simulink model "MATE_PermanentMagnetSynchronousMachine"  (R2024b)
settings: Solver=ode5  StartTime=0.0  StopTime=1  FixedStep=Ts_sim  MaxStep=Ts_sim  MinStep=Ts_sim / 100  RelTol=1e-3
PostLoadFcn:
  | Ts_sim=1e-6; Ts=Ts_sim;T_deadtime=5e-6;
  | PMSMDrive_Param;
InitFcn:
  | Ts_sim=1e-6; Ts=Ts_sim;T_deadtime=5e-6;
  | PMSMDrive_Param;
values from neighbouring files (symbols this model uses):
  carrier = 12000    [PMSMDrive_Param.m]
  inv_id_100 = 1 / id_100    [PMSMDrive_Param.m]
  inv_iq_100 = 1 / iq_100    [PMSMDrive_Param.m]
  inv_Kt = 1 / Kt    (= 1.0729615028)    [PMSMDrive_Param.m]
  iq_100 = Irms * sqrt3    [PMSMDrive_Param.m]
  iq_max = iq_100 * Torque_Lim / 100    [PMSMDrive_Param.m]
  Jall = J1 + J2    (= 0.0167309142)    [PMSMDrive_Param.m]
  Ld_100 = Ld / 1000    (= 0.002984)    [PMSMDrive_Param.m]
  Lq_100 = Lq / 1000    (= 0.004576)    [PMSMDrive_Param.m]
  Pm = Pole / 2    (= 3)    [PMSMDrive_Param.m]
  rad_to_rpm = 60 / 2 / pi    (= 9.54929658551)    [PMSMDrive_Param.m]
  rpm_to_rad = 1 / 60 * 2 * pi    (= 0.10471975512)    [PMSMDrive_Param.m]
  tr23 = sqrt23 * [ 1 0 ; -1/2 sqrt(3)/2 ; -1/2 -sqrt(3)/2 ]    [PMSMDrive_Param.m]
  tr32 = sqrt23 * [ 1 -1/2 -1/2 ; 0 sqrt(3)/2 -sqrt(3)/2 ]    [PMSMDrive_Param.m]
  Tsc = 50e-6    (= 5e-05)    [PMSMDrive_Param.m]
  V_upper = 400    [PMSMDrive_Param.m]
  VDC = 200 * sqrt(2)    [PMSMDrive_Param.m]
  wcc = 2000    [PMSMDrive_Param.m]
  wcpi = wcc / 10    (= 200)    [PMSMDrive_Param.m]
  wsc = 200    [PMSMDrive_Param.m]
  wspi = wsc / 10    (= 20)    [PMSMDrive_Param.m]
undefined symbols (not defined in the file or in its folder): DiscIntNeverNeededParam, PMSMDrive_Param, Vf
libraries: fl_lib x15, nesl_utility x13, simetranss x8, ee_lib x6, simulink x4
settings Model: ARTEMISmethode_block_infos=$$__separator__$$  Creator=Kyle Diller  LastModifiedBy=CD8435
settings SolverCC: AlgebraicLoopSolver=TrustRegion
settings DataIOCC: LimitDataPoints=on  SaveFormat=Array  SignalLoggingSaveFormat=ModelDataLogs  ReturnWorkspaceOutputs=off
settings OptimizationCC: ExpressionDepthLimit=2147483647  InitFltsAndDblsToZero=on  LifeSpan=inf
settings DebuggingCC: AlgebraicLoopMsg=error  ArtificialAlgebraicLoopMsg=error  SaveWithParameterizedLinksMsg=none  UnderspecifiedInitializationDetection=Classic  MergeDetectMultiDrivingBlocksExec=none  SignalResolutionControl=TryResolveAllWithWarning  SolverPrmCheckMsg=warning  MultiTaskDSMMsg=warning  MultiTaskCondExecSysMsg=none  FcnCallInpInsideContextMsg=warning  UnconnectedInputMsg=warning  UnconnectedOutputMsg=warning  UnconnectedLineMsg=warning  AllowSymbolicDim=off  StateNameClashWarn=warning  SFUnexpectedBacktrackingDiag=warning  SFNoUnconditionalDefaultTransitionDiag=warning  SFExecutionAtInitializationDiag=none  ArithmeticOperatorsInVariantConditions=warning
settings HardwareCC: ProdBitPerPointer=32  ProdBitPerSizeT=32  ProdBitPerPtrDiffT=32  ProdLargestAtomicFloat=None  ProdIntDivRoundTo=Undefined  ProdEndianess=Unspecified  ProdWordSize=32  ProdHWDeviceType=32-bit Generic
settings ModelReferenceCC: EnableRefExpFcnMdlSchedulingChecks=on  PropagateSignalLabelsOutOfModel=off
settings SFSimCC: SimUseLocalCustomCode=off  CustomCodeUndefinedFunction=UseInterfaceOnly
settings RTWCC: RTWUseLocalCustomCode=off  GPUComputeCapability=3.5
settings CodeAppCC: StateflowObjectComments=on
settings GRTTargetCC: TargetFcnLib=ansi_tfl_tmw.mat  TargetLangStandard=C89/C90 (ANSI)  CombineOutputUpdateFcns=off  GRTInterface=on
settings ConfigComp: CovMetricSettings=dw  CovSaveCumulativeToWorkspaceVar=on  CovSaveSingleToWorkspaceVar=on  CovExternalEMLEnable=off
settings SimscapeCC: SimscapeNormalizeSystem=off

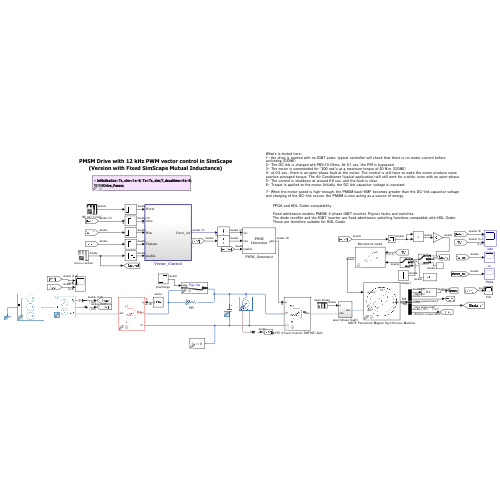
[thumbnail: Simulink's stored preview of the top-level diagram]
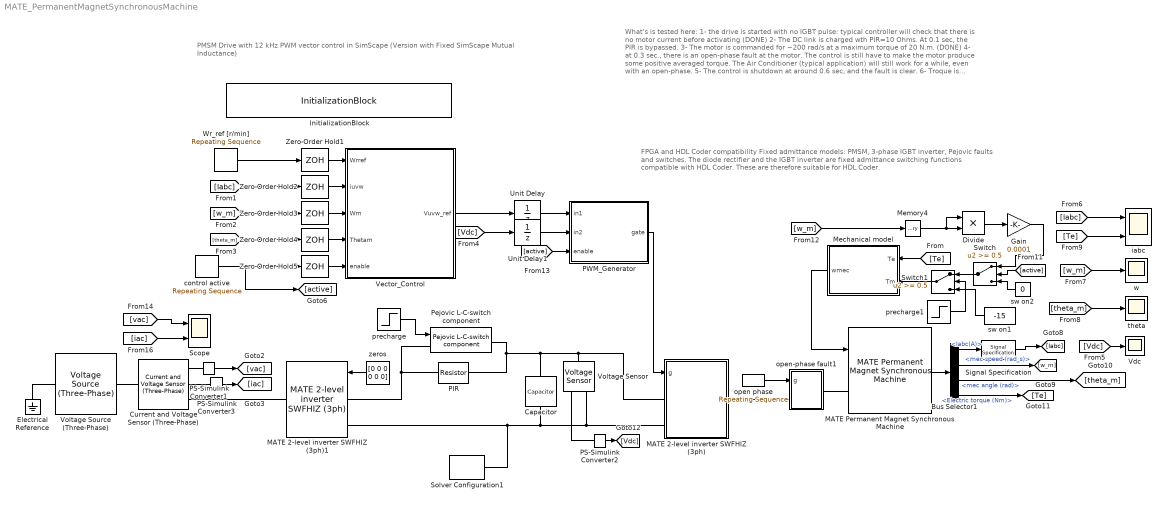
== system MATE_PermanentMagnetSynchronousMachine ==
  note: What's is tested here:
      | 1- the drive is started with no IGBT pulse: typical controller will check that there is no motor current before activating (DONE)
      | 2- The DC link is charged wth PIR=10 Ohms. At 0.1 sec, the PIR is bypassed.
      | 3- The motor is commanded for ~200 rad/s at a maximum torque of 20 N.m. (DONE)
      | 4- at 0.3 sec., there is an open-phase fault at the motor. The control is still have to make the motor produce some positive averaged torque. The Air Conditioner (typical application) will still work for a while, even with an open-phase.
      | 5- The control is shutdown at around 0.6 sec, and the fault is clear.
      | 6- Troque is applied to the motor. Initially, the DC link capacitor voltage is constant.
      |
      | 7- When the motor speed is high-enough, the PMSM back-EMF becomes greater than the DC-link capacitor voltage and charging of the DC-link occurs: the PMSM is now acting as a source of energy.
  note: PMSM Drive with 12 kHz PWM vector control in SimScape
      | (Version with Fixed SimScape Mutual Inductance)
  note: FPGA and HDL Coder compatibility
      |
      | Fixed admittance models: PMSM, 3-phase IGBT inverter, Pejovic faults and switches.
      | The diode rectifier and the IGBT inverter are fixed admittance switching functions compatible with HDL Coder.
      | These are therefore suitable for HDL Coder.
  Bus Selector1 : BusSelector  OutputSignals=Iabc(A),mec speed (rad_s),mec angle (rad),Electric torque (Nm)
  Capacitor : fl_lib/Electrical/Electrical Elements/Capacitor  c=1e-3 F  r=0 Ohm  g=0 1/Ohm  i_specify=off  i_priority=None  i=0 A  i_nominal_specify=off  i_nominal_value=1  i_nominal_unit=A  v_specify=off  v_priority=None  v=0 V  v_nominal_specify=off  v_nominal_value=1  v_nominal_unit=V  vc_specify=off  vc_priority=High  vc=0 V  vc_nominal_specify=off  vc_nominal_value=1  vc_nominal_unit=V
  Current and Voltage Sensor (Three-Phase) : ee_lib/Sensors & Transducers/Current and Voltage Sensor (Three-Phase)  vMeasurementType=ee.enum.vmeasurement.ll  outputUnit=ee.enum.unit.si  SRated=100e6 A*V  VRated=24e3 V  I_specify=off  I_priority=None  I=[0, 0, 0] A  I_nominal_specify=off  I_nominal_value=1  I_nominal_unit=A  V_specify=off  V_priority=None  V=[0, 0, 0] V  V_nominal_specify=off  V_nominal_value=1  V_nominal_unit=V
      settings: InternalSimscapePortConfiguration="{\"Bottom\":[],\"Left\":[{\"id\":\"N1\",\"label\":\"~1\",\"type\":\"foundation.electrical.three_phase\"}],\"Right\":[{\"id\":\"V_output\",\"label\":\"V\",\"type\":\"output\"},{\"id\":\"I_output\",\"label\":\"I\",\"type\":\"output\"},{\"id\":\"N2\",\"label\":\"~2\",\"type\":\"foundation.electrical.three_phase\"}],\"Top\":[]}"
  Divide : Product
  Electrical Reference : fl_lib/Electrical/Electrical Elements/Electrical Reference
  Gain : Gain  Gain=0.0001
  InitializationBlock : simetranss/Usefulls/InitializationBlock  InitVar=Ts_sim=1e-6; Ts=Ts_sim;T_deadtime=5e-6;  InitFile=PMSMDrive_Param;  prel=off  posl=on  inif=on
  MATE 2-level inverter SWFHIZ (3ph) : Subsystem  AncestorBlock=simetranss/FPGA/MATE 2-level inverter SWFHIZ (3ph)  mask(MATE Inverter Switching Function (2-level IGBT/Diode) (3-phase)){Ron=1e-3, Gpp=250, Gip=0.1e-6, Ts=Ts, min_charge=0.1}
      mask prompts: Ron "Switch Ron (Ohms)"; Gpp "Snubber resistance (Ohms)"; Gip "Snubber Capacitor (Ohms)"; Ts "Sample time (s)"; min_charge "Minimum rectifying current (A)"
      mask help:
      | This block implements a 3-phase  2-level inverter as a switching function.
      |
      | The block is Time-Step-Averaging-capable meaning that the averaging gate ON-time is averaged at each time step.
      |
      | With this approach, dead-times smaller than the sample time are accurately taken into account.
      |
      | The inverter can be in high impedance and rectifying states by selecting correctly the RC snubber.
      | Typically Rsnubber=L_load/Ts , then adjust Csnubber so Rsnubber*Csnubber=2*Ts.
      |
      | Minimum Rectifying current: In passive mode (no IGBT pulsing), this is the minimum rectifying current that is injected to the DC bus. This parameter is used to avoid unrealistic DC-bus charging when the inverter acts as a diode recfifier and do not impact in active control (gate pulsing) mode.
      |
      | The block has a constant admittance and is suitable for HDL coder.
  MATE 2-level inverter SWFHIZ (3ph)1 : simetranss/FPGA/MATE 2-level inverter SWFHIZ (3ph)  Ron=1e-3  Vf=0  Gpp=250  Gip=0.1e-6  Ts=Ts  min_charge=0.1
  MATE Permanent Magnet Synchronous Machine : simetranss/Machines/MATE Permanent Magnet Synchronous Machine  Rs=0.12  rtyp=Salient (Ld != Lq)  Ld=0.002984  Lq=0.004576  Ldd=0.003  Mf=0.25366  pp=3  AngInit=0  sal_der=0.1  Ts=Ts
  Mechanical model : Subsystem  mask(Machine rotational mechanical model){J=0.016731, F=0, fo=0, Ts=Ts}
      mask prompts: J "Inertia (kg.m^2)"; F "Friction (N.m.s)"; fo "Initial mechanical frequency (Hz)"; Ts "Sample Time (s)"
      mask help:
      | This block can implement the mechanical equation of rotating machines.
      |
      | The block working equation is:
      | wmec=1/J*INTEGRAL{( Te - Tm -F*wmec )*dt}
      |
      | All values in SI.
      |
      | Parameters:
      | Inertia J (kg.m^2)
      | Friction F (N.m.s)
      | Initial mechanical frequency (Hz)
      | Sample Time (s).
      |
      | Signals:
      | Te: electric torque input from the machine (N.m.)
      | Tm : mechanical torque applied to the shaft (N.m.)
      | wmec: mechanical speed of machine (rad/s)
      |
      | Conversion from Per-Unit values
      |
      | J=2*H*Pn/w_mec^2
      | F=D*Pn/w_mec^2
      | where:
      | J is the inertia in km.m^2
      | H is the inertia constant in seconds.
      | F is the friction factor in N.m.s
      | D in the friction factor or damping factor in pu.
      | Pn is the nominal power of the machine
      | w_mec is the nominal mechanical rotational frequency of the machine in rad/s
  Memory4 : Memory  InheritSampleTime=on
  PIR : fl_lib/Electrical/Electrical Elements/Resistor  R=10 Ohm  i_specify=off  i_priority=None  i=0 A  i_nominal_specify=off  i_nominal_value=1  i_nominal_unit=A  v_specify=off  v_priority=None  v=0 V  v_nominal_specify=off  v_nominal_value=1  v_nominal_unit=V
  PS-Simulink Converter1 : nesl_utility/PS-Simulink Converter  PhysicalDomain=network_engine_domain  SubClassName=ps_output  LeftPortType=input  RightPortType=output  PseudoPeriodic=off  Frequencies=[]  VectorFormat=inherit  Unit=inherit  AffineConversion=off
  PS-Simulink Converter2 : nesl_utility/PS-Simulink Converter  PhysicalDomain=network_engine_domain  SubClassName=ps_output  LeftPortType=input  RightPortType=output  PseudoPeriodic=off  Frequencies=[]  VectorFormat=inherit  Unit=inherit  AffineConversion=off
  PS-Simulink Converter3 : nesl_utility/PS-Simulink Converter  PhysicalDomain=network_engine_domain  SubClassName=ps_output  LeftPortType=input  RightPortType=output  PseudoPeriodic=off  Frequencies=[]  VectorFormat=inherit  Unit=inherit  AffineConversion=off
  PWM_Generator : Subsystem
      mask Display: disp(' PWM \n Generator ')
  Pejovic L-C-switch component : simetranss/FPGA/Pejovic L-C-switch component  typ=Switch  Lon=1e-7  L=100e-6  C=300e-9  traprule=off  otherSW='coming soon'  Ts=Ts  pcbp=off  showV=off  showI=off
  Scope : Scope  NumInputPorts=2
  Signal Specification : SignalSpecification  Dimensions=3
  Solver Configuration1 : nesl_utility/Solver Configuration  PhysicalDomain=network_engine_domain  SubClassName=solver  LeftPortType=input  RightPortType=generic  Tones=[]  Harmonics=[]  SimulateNoise=off  Profile=off  UseLocalSampling=off  EnableSwitchedLinearOptims=on  FrequencyDomain=off  UseCCode=off  RelTol=0.001  AbsTol=1e-06  MinStep=1e-09  ToWorkspace=off  RevertToSquareIcSolve=off  NumHomotopyIterations=100  PhasorMode=off  PhasorModeNumHarmonics=1  ConsistencySolver=NEWTON_FTOL  IndexReductionMethod=DerivativeReplacement  DoDC=off  ResidualTolerance=0.001  ConsistencyTolSource=GLOBAL  ConsistencyAbsTol=0.001  ConsistencyRelTol=0.001  ConsistencyTolFactor=0.001  UseLocalSolver=on  LocalSolverChoice=NE_BACKWARD_EULER_ADVANCER  ResolveIndetEquations=off  FunctionEvalNumThread=1  LocalSolverSampleTime=Ts  DoFixedCost=on  MaxNonlinIter=1  MaxModeIter=2  ComputeImpulses=off  ImpulseIterations=2  LinearAlgebra=Sparse  LinearAlgebraNumThread=0  EquationFormulation=NE_TIME_EF  DelaysMemoryBudget=1024  AutomaticFiltering=off  FilteringTimeConstant=0.001  PartitionStorageMethod=AS_NEEDED  PartitionMemoryBudget=1024  PartitionMethod=ROBUST  MultibodyUseLocalSolver=off  MultibodyLocalSolverChoice=ODE1  MultibodyLocalSolverSampleTime=0.001
  Switch : Switch  Threshold=0.5  SaturateOnIntegerOverflow=off  InputSameDT=off
  Switch1 : Switch  Threshold=0.5  SaturateOnIntegerOverflow=off  InputSameDT=off
  Unit Delay : UnitDelay  SampleTime=Ts  HasFrameUpgradeWarning=on
  Unit Delay1 : UnitDelay  SampleTime=Ts  HasFrameUpgradeWarning=on
  Vdc : Scope
  Vector_Control : Subsystem  TreatAsAtomicUnit=on
  Voltage Source (Three-Phase) : ee_lib/Sources/Voltage Source (Three-Phase)  vline_rms=200 V  shift=0 deg  freq=60 Hz  impedance_option=4  SShortCircuit=10000e6 A*V  XR=15  R=0.011 Ohm  L=1e-4 H  harmonic_option=0  harmonic_orders=[5, 7, 11, 13]  harmonic_ratios=[.1, .1, .1, .1]  G_parasitic=0 1/Ohm  I_specify=on  I_priority=High  I=[0, 0, 0] A  I_nominal_specify=off  I_nominal_value=1  I_nominal_unit=A
  Voltage Sensor : fl_lib/Electrical/Electrical Sensors/Voltage Sensor
  Wr_ref [r/min] : simulink/Sources/Repeating Sequence  rep_seq_t=[ 0 0.1 0.1+eps 0.15 0.15+eps 0.6]  rep_seq_y=[ 0 0 1000 1000 2000 2000] * rpm_to_rad
  Zero-Order Hold{1..5} (5 alike) : ZeroOrderHold  SampleTime=Tsc
  control active : simulink/Sources/Repeating Sequence  rep_seq_t="[ 0 0.09 0.09+Ts  0.6 0.6+Ts  2]"  rep_seq_y=[ 0 0 1 1 0 0]
  iabc : Scope  NumInputPorts=2
  open phase : simulink/Sources/Repeating Sequence  rep_seq_t="[ 0 0.4 0.4+Ts  0.6 0.6+Ts  2]"  rep_seq_y=[ 1 1 0 0 1 1]
  open-phase fault1 : Subsystem
  precharge : Step  Time=0.1  SampleTime=0
  precharge1 : Step  Time=0.7  Before=1  After=0  SampleTime=0
  sw on1 : Constant  Value=-15
  sw on2 : Constant  Value=0
  theta : Scope
  w : Scope
  zeros : Constant  Value=[0 0 0 0 0 0]
  wires:
  [theta_m] -> Zero-Order Hold4/1
  [w_m] -> Zero-Order Hold3/1
  [Iabc] -> Zero-Order Hold2/1
  [w_m] -> Memory4/1
  Wr_ref [r/min]/1 -> Zero-Order Hold1/1
  Vector_Control/1(Vuvw_ref) -> Unit Delay/1
  [Vdc] -> Unit Delay1/1
  [Vdc] -> Vdc/1
  [Iabc] -> iabc/1
  [w_m] -> w/1
  [theta_m] -> theta/1
  [Te] -> iabc/2
  control active/1 -> [active], Zero-Order Hold5/1
  [active] -> Switch/2
  [active] -> PWM_Generator/3(enable)
  [Te] -> Mechanical model/1(Te)
  PWM_Generator/1(gate) -> MATE 2-level inverter SWFHIZ (3ph)/1(g)
  Bus Selector1/3 -> [theta_m]  "<mec angle (rad)>"
  Bus Selector1/2 -> [w_m]  "<mec speed (rad_s)>"
  Bus Selector1/4 -> [Te]  "<Electric torque (Nm)>"
  Bus Selector1/1 -> Signal Specification/1  "<Iabc(A)>"
  PS-Simulink Converter2/1 -> [Vdc]
  Zero-Order Hold1/1 -> Vector_Control/1(Wrref)
  Zero-Order Hold2/1 -> Vector_Control/2(iuvw)
  Zero-Order Hold3/1 -> Vector_Control/3(Wm)
  Zero-Order Hold4/1 -> Vector_Control/4(Thetam)
  Zero-Order Hold5/1 -> Vector_Control/5(enable)
  Unit Delay/1 -> PWM_Generator/1(in1)
  open phase/1 -> open-phase fault1/1(g)
  precharge/1 -> Pejovic L-C-switch component/1
  Mechanical model/1(wmec) -> MATE Permanent Magnet Synchronous Machine/1
  sw on1/1 -> Switch1/3
  precharge1/1 -> Switch1/2
  Unit Delay1/1 -> PWM_Generator/2(in2)
  PS-Simulink Converter1/1 -> [vac]
  PS-Simulink Converter3/1 -> [iac]
  [vac] -> Scope/1
  [iac] -> Scope/2
  sw on2/1 -> Switch/3
  Memory4/1 -> Divide/1, Divide/2
  Divide/1 -> Gain/1
  Gain/1 -> Switch/1
  zeros/1 -> MATE 2-level inverter SWFHIZ (3ph)1/1
  Switch1/1 -> Mechanical model/2(Tm)
  Switch/1 -> Switch1/1
  Signal Specification/1 -> [Iabc]
  MATE Permanent Magnet Synchronous Machine/1 -> Bus Selector1/1
  connections:
  Electrical Reference/LConn1 -- Voltage Source (Three-Phase)/LConn1
  Pejovic L-C-switch component/RConn1 -- PIR/RConn1 -- Capacitor/LConn1 -- Voltage Sensor/LConn1 -- MATE 2-level inverter SWFHIZ (3ph)/LConn1
  Capacitor/RConn1 -- Voltage Sensor/RConn2 -- MATE 2-level inverter SWFHIZ (3ph)/LConn2 -- Solver Configuration1/RConn1 -- MATE 2-level inverter SWFHIZ (3ph)1/LConn2
  Voltage Sensor/RConn1 -- PS-Simulink Converter2/LConn1
  Voltage Source (Three-Phase)/RConn1 -- Current and Voltage Sensor (Three-Phase)/LConn1
  MATE 2-level inverter SWFHIZ (3ph)1/RConn1 -- Current and Voltage Sensor (Three-Phase)/RConn3
  PS-Simulink Converter1/LConn1 -- Current and Voltage Sensor (Three-Phase)/RConn1
  Current and Voltage Sensor (Three-Phase)/RConn2 -- PS-Simulink Converter3/LConn1
  MATE 2-level inverter SWFHIZ (3ph)1/LConn1 -- PIR/LConn1 -- Pejovic L-C-switch component/LConn1
  MATE Permanent Magnet Synchronous Machine/LConn1 -- open-phase fault1/RConn1
  MATE 2-level inverter SWFHIZ (3ph)/RConn1 -- open-phase fault1/LConn1

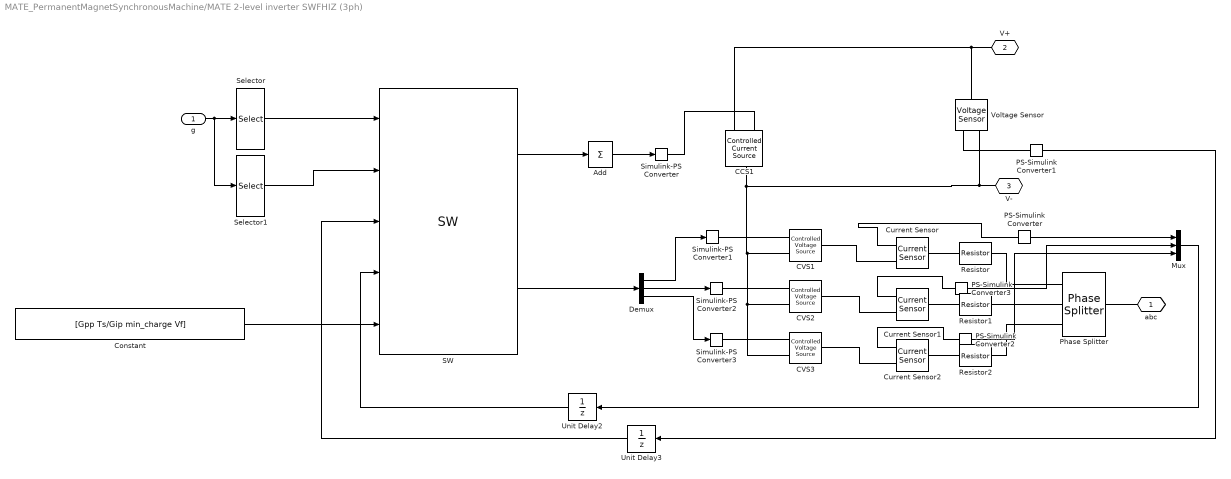
== system MATE_PermanentMagnetSynchronousMachine/MATE 2-level inverter SWFHIZ (3ph) ==
  g : Inport
  Add : Sum  Inputs=+
  CCS1 : fl_lib/Electrical/Electrical Sources/Controlled Current Source
  CVS1 : fl_lib/Electrical/Electrical Sources/Controlled Voltage Source
  CVS2 : fl_lib/Electrical/Electrical Sources/Controlled Voltage Source
  CVS3 : fl_lib/Electrical/Electrical Sources/Controlled Voltage Source
  Constant : Constant  Value=[Gpp Ts/Gip min_charge Vf]
  Current Sensor : fl_lib/Electrical/Electrical Sensors/Current Sensor
  Current Sensor1 : fl_lib/Electrical/Electrical Sensors/Current Sensor
  Current Sensor2 : fl_lib/Electrical/Electrical Sensors/Current Sensor
  Demux : Demux  Outputs=3
  Mux : Mux  Inputs=3
  PS-Simulink Converter{,1..3} (4 alike) : nesl_utility/PS-Simulink Converter  PhysicalDomain=network_engine_domain  SubClassName=ps_output  LeftPortType=input  RightPortType=output  PseudoPeriodic=off  Frequencies=[]  VectorFormat=inherit  Unit=inherit  AffineConversion=off
  Phase Splitter : ee_lib/Connectors & References/Phase Splitter
  Resistor : fl_lib/Electrical/Electrical Elements/Resistor  R=Ron Ohm  i_specify=off  i_priority=None  i=0 A  i_nominal_specify=off  i_nominal_value=1  i_nominal_unit=A  v_specify=off  v_priority=None  v=0 V  v_nominal_specify=off  v_nominal_value=1  v_nominal_unit=V
  Resistor1 : fl_lib/Electrical/Electrical Elements/Resistor  R=Ron Ohm  i_specify=off  i_priority=None  i=0 A  i_nominal_specify=off  i_nominal_value=1  i_nominal_unit=A  v_specify=off  v_priority=None  v=0 V  v_nominal_specify=off  v_nominal_value=1  v_nominal_unit=V
  Resistor2 : fl_lib/Electrical/Electrical Elements/Resistor  R=Ron Ohm  i_specify=off  i_priority=None  i=0 A  i_nominal_specify=off  i_nominal_value=1  i_nominal_unit=A  v_specify=off  v_priority=None  v=0 V  v_nominal_specify=off  v_nominal_value=1  v_nominal_unit=V
  SW : simetranss/FPGA/MATE 2-level inverter SWFHIZ/SW  SystemSampleTime=-1  VariantActivationTime=update diagram  AllowFlexibleInterface=on  Latency=0  AutoFrameSizeCalculation=off
  Selector : Selector  InputPortWidth=6  IndexOptions=Index vector (dialog)  Indices=[1 3 5]  OutputSizes=1
  Selector1 : Selector  InputPortWidth=6  IndexOptions=Index vector (dialog)  Indices=[1 3 5]+1  OutputSizes=1
  Simulink-PS Converter{,1..3} (4 alike) : nesl_utility/Simulink-PS Converter  PhysicalDomain=network_engine_domain  SubClassName=ps_input  LeftPortType=input  RightPortType=output  PseudoPeriodic=off  Frequencies=[]  NoiseDistribution=none  NoiseParameters=[]  Unit=1  AffineConversion=off  FilteringAndDerivatives=provide  SimscapeFilterOrder=1  InputFilterTimeConstant=0.001  UdotUserProvided=0
  Unit Delay2 : UnitDelay  SampleTime=Ts  HasFrameUpgradeWarning=on
  Unit Delay3 : UnitDelay  SampleTime=Ts  HasFrameUpgradeWarning=on
  Voltage Sensor : fl_lib/Electrical/Electrical Sensors/Voltage Sensor
  abc : PMIOPort  Side=Right
  V+ : PMIOPort  Port=2  Side=Left
  V- : PMIOPort  Port=3  Side=Left
  wires:
  Add/1 -> Simulink-PS Converter/1
  g/1 -> Selector1/1, Selector/1
  SW/1 -> Add/1
  PS-Simulink Converter/1 -> Mux/1
  PS-Simulink Converter3/1 -> Mux/2
  PS-Simulink Converter2/1 -> Mux/3
  Demux/3 -> Simulink-PS Converter3/1
  Demux/2 -> Simulink-PS Converter2/1
  Demux/1 -> Simulink-PS Converter1/1
  SW/2 -> Demux/1
  Selector/1 -> SW/1
  Selector1/1 -> SW/2
  Constant/1 -> SW/5
  PS-Simulink Converter1/1 -> Unit Delay3/1
  Mux/1 -> Unit Delay2/1
  Unit Delay2/1 -> SW/4
  Unit Delay3/1 -> SW/3
  connections:
  Simulink-PS Converter/RConn1 -- CCS1/RConn1
  PS-Simulink Converter/LConn1 -- Current Sensor/RConn1
  Simulink-PS Converter1/RConn1 -- CVS1/RConn1
  CVS1/RConn2 -- V-/RConn1 -- Voltage Sensor/RConn2 -- CCS1/LConn1 -- CVS2/RConn2 -- CVS3/RConn2
  CCS1/RConn2 -- V+/RConn1 -- Voltage Sensor/LConn1
  PS-Simulink Converter1/LConn1 -- Voltage Sensor/RConn1
  Phase Splitter/LConn1 -- abc/RConn1
  Resistor/RConn1 -- Phase Splitter/RConn1
  Resistor1/RConn1 -- Phase Splitter/RConn2
  Resistor2/RConn1 -- Phase Splitter/RConn3
  PS-Simulink Converter3/LConn1 -- Current Sensor1/RConn1
  PS-Simulink Converter2/LConn1 -- Current Sensor2/RConn1
  Simulink-PS Converter2/RConn1 -- CVS2/RConn1
  Simulink-PS Converter3/RConn1 -- CVS3/RConn1
  CVS1/LConn1 -- Current Sensor/RConn2
  CVS2/LConn1 -- Current Sensor1/RConn2
  CVS3/LConn1 -- Current Sensor2/RConn2
  Current Sensor2/LConn1 -- Resistor2/LConn1
  Current Sensor1/LConn1 -- Resistor1/LConn1
  Current Sensor/LConn1 -- Resistor/LConn1

== system MATE_PermanentMagnetSynchronousMachine/Mechanical model ==
  note: Pm=Tm*w so a divider by w can be added if Pm is provided instead of Tm
  Te : Inport  PortDimensions=1
  Tm : Inport  Port=2
  1 ----- J : Gain  Gain=1/J  SaturateOnIntegerOverflow=on  OutDataTypeStr=Inherit: Same as input  ParamDataTypeStr=Inherit: Same as input
  F : Gain  Gain=F  SaturateOnIntegerOverflow=on  OutDataTypeStr=Inherit: Same as input  ParamDataTypeStr=Inherit: Same as input
  Rotor speed interator : DiscreteIntegrator  InitialCondition=fo*2*pi  SampleTime=Ts  ICPrevOutput=DiscIntNeverNeededParam  ICPrevScaledInput=DiscIntNeverNeededParam
  Sum2 : Sum  Inputs=-+-  InputSameDT=on  SaturateOnIntegerOverflow=on  OutDataTypeStr=Inherit: Same as first input
  wmec : Outport  InitialOutput=0  VectorParamsAs1DForOutWhenUnconnected=off
  wires:
  Tm/1 -> Sum2/1  "Tm"
  Sum2/1 -> 1 ----- J/1
  F/1 -> Sum2/3
  Te/1 -> Sum2/2  "Te"
  1 ----- J/1 -> Rotor speed interator/1
  Rotor speed interator/1 -> wmec/1, F/1  "w"

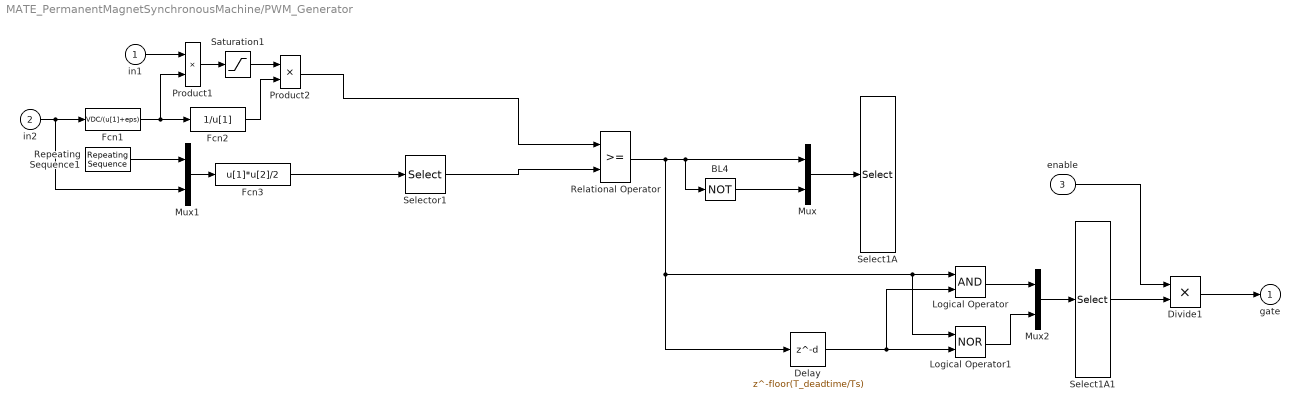
== system MATE_PermanentMagnetSynchronousMachine/PWM_Generator ==
  in1 : Inport
  in2 : Inport  Port=2
  enable : Inport  Port=3
  BL4 : Logic  Operator=NOT  Inputs=1
  Delay : Delay  DelayLength=floor(T_deadtime/Ts)
  Divide1 : Product
  Fcn1 : Fcn  Expr=VDC/(u[1]+eps)
  Fcn2 : Fcn  Expr=1/u[1]
  Fcn3 : Fcn  Expr=u[1]*u[2]/2
  Logical Operator : Logic  AllPortsSameDT=off  OutDataTypeStr=boolean
  Logical Operator1 : Logic  Operator=NOR  AllPortsSameDT=off  OutDataTypeStr=boolean
  Mux : Mux  Inputs=2
  Mux1 : Mux  Inputs=2
  Mux2 : Mux  Inputs=2
  Product1 : Product  InputSameDT=on  SaturateOnIntegerOverflow=on  OutDataTypeStr=Inherit: Same as first input
  Product2 : Product  InputSameDT=on  SaturateOnIntegerOverflow=on  OutDataTypeStr=Inherit: Same as first input
  Relational Operator : RelationalOperator
  Repeating Sequence1 : simulink/Sources/Repeating Sequence  rep_seq_t=[ 0 1/carrier/2 1/carrier ]  rep_seq_y=[ -1 1 -1 ]
  Saturation1 : Saturate  UpperLimit=VDC/2  LowerLimit=-VDC/2
  Select1A : Selector  InputPortWidth=6  IndexOptions=Index vector (dialog)  Indices=[1 4 2 5 3 6]  OutputSizes=1
  Select1A1 : Selector  InputPortWidth=6  IndexOptions=Index vector (dialog)  Indices=[1 4 2 5 3 6]  OutputSizes=1
  Selector1 : Selector  InputPortWidth=1  IndexOptions=Index vector (dialog)  Indices=[1 1 1]  OutputSizes=1
  gate : Outport  VectorParamsAs1DForOutWhenUnconnected=off
  wires:
  Selector1/1 -> Relational Operator/2
  Repeating Sequence1/1 -> Mux1/1
  Mux1/1 -> Fcn3/1
  Fcn2/1 -> Product2/2
  Saturation1/1 -> Product2/1
  Product1/1 -> Saturation1/1
  Fcn1/1 -> Fcn2/1, Product1/2
  in1/1 -> Product1/1
  Product2/1 -> Relational Operator/1
  in2/1 -> Fcn1/1, Mux1/2
  Fcn3/1 -> Selector1/1
  Relational Operator/1 -> Delay/1, Logical Operator1/1, Logical Operator/1, BL4/1, Mux/1
  BL4/1 -> Mux/2
  Mux/1 -> Select1A/1
  enable/1 -> Divide1/1
  Delay/1 -> Logical Operator/2, Logical Operator1/2
  Logical Operator/1 -> Mux2/1
  Logical Operator1/1 -> Mux2/2
  Mux2/1 -> Select1A1/1
  Select1A1/1 -> Divide1/2
  Divide1/1 -> gate/1

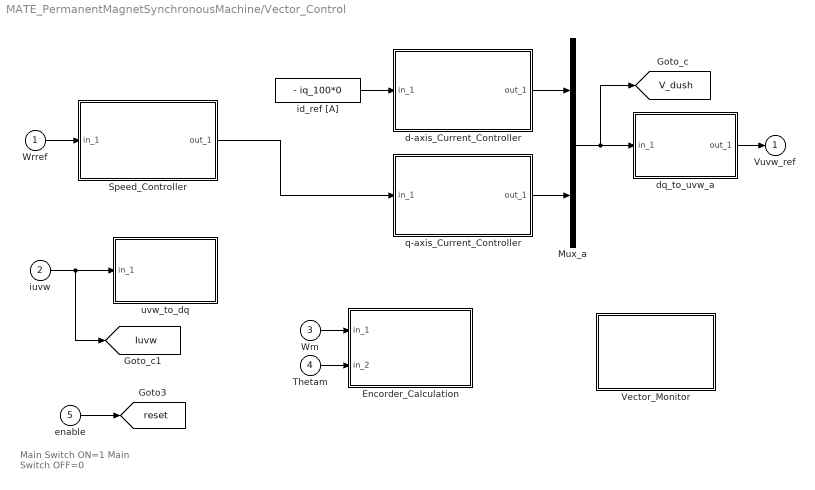
== system MATE_PermanentMagnetSynchronousMachine/Vector_Control ==
  note: Main Switch ON=1
      | Main Switch OFF=0
  Wrref : Inport
  iuvw : Inport  Port=2
  Wm : Inport  Port=3
  Thetam : Inport  Port=4
  enable : Inport  Port=5
  Encorder_Calculation : Subsystem
      mask Display: disp(' Encorder \n Calculation ')
  Mux_a : Mux  Inputs=2
  Speed_Controller : Subsystem
      mask Display: disp(' Speed \n Controller ')
  Vector_Monitor : Subsystem
      mask Display:
      | plot([0,1],[0,0])
      | plot([0,1],[1,1])
      | disp(' Vector \n Monitor ')
  d-axis_Current_Controller : Subsystem
      mask Display: disp(' Current \n Controller ')
  dq_to_uvw_a : Subsystem
      mask Display: disp(' Coordinate \n Transform')
  id_ref [A] : Constant  Value=- iq_100*0
  q-axis_Current_Controller : Subsystem
      mask Display: disp(' Current \n Controller ')
  uvw_to_dq : Subsystem
      mask Display: disp(' Coordinate \n Transform ')
  Vuvw_ref : Outport  InitialOutput=0
  tag scope: Iuvw=global, V_dush=global, reset=global
  wires:
  Wrref/1 -> Speed_Controller/1(in_1)
  Wm/1 -> Encorder_Calculation/1(in_1)
  iuvw/1 -> uvw_to_dq/1(in_1), [Iuvw]
  q-axis_Current_Controller/1(out_1) -> Mux_a/2
  d-axis_Current_Controller/1(out_1) -> Mux_a/1
  Mux_a/1 -> dq_to_uvw_a/1(in_1), [V_dush]
  dq_to_uvw_a/1(out_1) -> Vuvw_ref/1
  Thetam/1 -> Encorder_Calculation/2(in_2)
  enable/1 -> [reset]
  Speed_Controller/1(out_1) -> q-axis_Current_Controller/1(in_1)
  id_ref [A]/1 -> d-axis_Current_Controller/1(in_1)

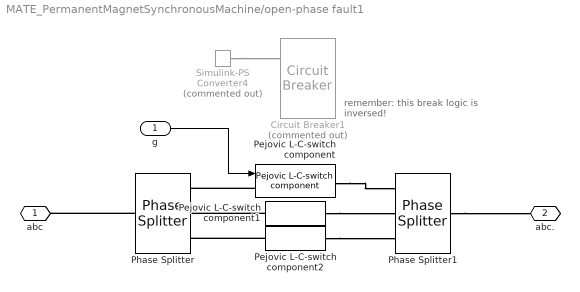
== system MATE_PermanentMagnetSynchronousMachine/open-phase fault1 ==
  note: remember: this break logic is inversed!
  g : Inport
  Circuit Breaker1 : ee_lib/Switches & Breakers/Circuit Breaker  Commented=on  R_closed=0.01 Ohm  G_open=1e-6 1/Ohm  threshold=0.5 V  breaker_behavior=ee.enum.switches.breakerBehavior.zeroCrossingDisable
      settings: InternalSimscapePortConfiguration="{\"Bottom\":[],\"Left\":[{\"id\":\"vT\",\"label\":\"vT\",\"type\":\"input\"},{\"id\":\"p1\",\"label\":\"\",\"type\":\"foundation.electrical.electrical\"}],\"Right\":[{\"id\":\"p2\",\"label\":\"\",\"type\":\"foundation.electrical.electrical\"}],\"Top\":[]}"
  Pejovic L-C-switch component : simetranss/FPGA/Pejovic L-C-switch component  typ=Switch  Lon=1e-7  L=100e-6  C=300e-9  traprule=off  otherSW='coming soon'  Ts=Ts  pcbp=off  showV=off  showI=off
  Pejovic L-C-switch component1 : simetranss/FPGA/Pejovic L-C-switch component  typ=Inductor  Lon=1e-7  L=1e-7  C=300e-9  traprule=off  otherSW='coming soon'  Ts=Ts  pcbp=off  showV=off  showI=off
  Pejovic L-C-switch component2 : simetranss/FPGA/Pejovic L-C-switch component  typ=Inductor  Lon=1e-7  L=1e-7  C=300e-9  traprule=off  otherSW='coming soon'  Ts=Ts  pcbp=off  showV=off  showI=off
  Phase Splitter : ee_lib/Connectors & References/Phase Splitter
  Phase Splitter1 : ee_lib/Connectors & References/Phase Splitter
  Simulink-PS Converter4 : nesl_utility/Simulink-PS Converter  Commented=on  PhysicalDomain=network_engine_domain  SubClassName=ps_input  LeftPortType=input  RightPortType=output  PseudoPeriodic=off  Frequencies=[]  NoiseDistribution=none  NoiseParameters=[]  Unit=1  AffineConversion=off  FilteringAndDerivatives=provide  SimscapeFilterOrder=1  InputFilterTimeConstant=0.001  UdotUserProvided=0
  abc : PMIOPort  Side=Left
  abc. : PMIOPort  Port=2  Side=Right
  wires:
  g/1 -> Pejovic L-C-switch component/1
  connections:
  Pejovic L-C-switch component2/RConn1 -- Phase Splitter1/RConn3
  Pejovic L-C-switch component1/RConn1 -- Phase Splitter1/RConn2
  Simulink-PS Converter4/RConn1 -- Circuit Breaker1/LConn1
  Phase Splitter1/LConn1 -- abc./RConn1
  Pejovic L-C-switch component1/LConn1 -- Phase Splitter/RConn2
  Phase Splitter/LConn1 -- abc/RConn1
  Pejovic L-C-switch component/RConn1 -- Phase Splitter1/RConn1
  Pejovic L-C-switch component2/LConn1 -- Phase Splitter/RConn3
  Pejovic L-C-switch component/LConn1 -- Phase Splitter/RConn1

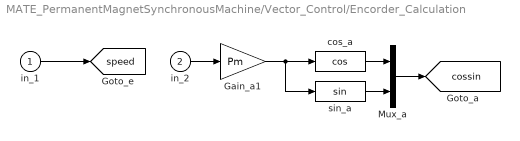
== system MATE_PermanentMagnetSynchronousMachine/Vector_Control/Encorder_Calculation ==
  in_1 : Inport
  in_2 : Inport  Port=2
  Gain_a1 : Gain  Gain=Pm  SaturateOnIntegerOverflow=on  OutDataTypeStr=Inherit: Same as input  ParamDataTypeStr=Inherit: Same as input
  Mux_a : Mux  Inputs=2
  cos_a : Trigonometry  Operator=cos
  sin_a : Trigonometry
  tag scope: cossin=global, speed=global
  wires:
  Mux_a/1 -> [cossin]
  sin_a/1 -> Mux_a/2
  cos_a/1 -> Mux_a/1
  in_2/1 -> Gain_a1/1
  in_1/1 -> [speed]
  Gain_a1/1 -> cos_a/1, sin_a/1

== system MATE_PermanentMagnetSynchronousMachine/Vector_Control/Speed_Controller ==
  in_1 : Inport
  PI_Controller : Subsystem
      mask Display: disp(' PI \n Controller ')
  error : Subsystem
      mask Display: disp('err')
  out_1 : Outport
  wires:
  error/1(out_1) -> PI_Controller/1(in_1)
  PI_Controller/1(out_1) -> out_1/1
  in_1/1 -> error/1(in_1)
  [speed] -> error/2(in_2)

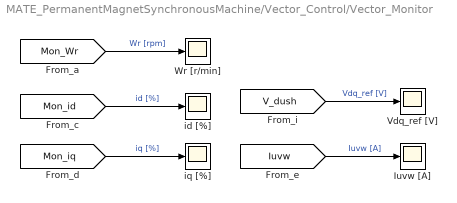
== system MATE_PermanentMagnetSynchronousMachine/Vector_Control/Vector_Monitor ==
  Iuvw [A] : Scope
  Vdq_ref [V] : Scope
  Wr [r/min] : Scope
  id [%] : Scope
  iq [%] : Scope
  wires:
  [Mon_iq] -> iq [%]/1  "iq [%]"
  [Mon_id] -> id [%]/1  "id [%]"
  [Mon_Wr] -> Wr [r/min]/1  "Wr [rpm]"
  [Iuvw] -> Iuvw [A]/1  "Iuvw [A]"
  [V_dush] -> Vdq_ref [V]/1  "Vdq_ref [V]"

== system MATE_PermanentMagnetSynchronousMachine/Vector_Control/d-axis_Current_Controller ==
  in_1 : Inport
  PI_Controller : Subsystem
      mask Display: disp(' PI \n Controller ')
  error : Subsystem
      mask Display: disp('err')
  out_1 : Outport
  wires:
  error/1(out_1) -> PI_Controller/1(in_1)
  PI_Controller/1(out_1) -> out_1/1
  in_1/1 -> error/1(in_1)
  [id_FB] -> error/2(in_2)

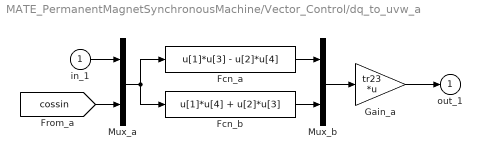
== system MATE_PermanentMagnetSynchronousMachine/Vector_Control/dq_to_uvw_a ==
  in_1 : Inport
  Fcn_a : Fcn  Expr=u[1]*u[3] - u[2]*u[4]
  Fcn_b : Fcn  Expr=u[1]*u[4] + u[2]*u[3]
  Gain_a : Gain  Gain=tr23  Multiplication=Matrix(K*u)  SaturateOnIntegerOverflow=on  OutDataTypeStr=Inherit: Same as input  ParamDataTypeStr=Inherit: Same as input
  Mux_a : Mux  Inputs=2
  Mux_b : Mux  Inputs=2
  out_1 : Outport
  wires:
  Mux_b/1 -> Gain_a/1
  Fcn_b/1 -> Mux_b/2
  Fcn_a/1 -> Mux_b/1
  Gain_a/1 -> out_1/1
  in_1/1 -> Mux_a/1
  [cossin] -> Mux_a/2
  Mux_a/1 -> Fcn_a/1, Fcn_b/1

== system MATE_PermanentMagnetSynchronousMachine/Vector_Control/q-axis_Current_Controller ==
  in_1 : Inport
  PI_Controller : Subsystem
      mask Display: disp(' PI \n Controller ')
  error : Subsystem
      mask Display: disp('err')
  out_1 : Outport
  wires:
  [iq_FB] -> error/2(in_2)
  in_1/1 -> error/1(in_1)
  PI_Controller/1(out_1) -> out_1/1
  error/1(out_1) -> PI_Controller/1(in_1)

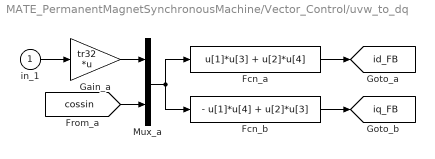
== system MATE_PermanentMagnetSynchronousMachine/Vector_Control/uvw_to_dq ==
  in_1 : Inport
  Fcn_a : Fcn  Expr=u[1]*u[3] + u[2]*u[4]
  Fcn_b : Fcn  Expr=- u[1]*u[4] + u[2]*u[3]
  Gain_a : Gain  Gain=tr32  Multiplication=Matrix(K*u)  SaturateOnIntegerOverflow=on  OutDataTypeStr=Inherit: Same as input  ParamDataTypeStr=Inherit: Same as input
  Mux_a : Mux  Inputs=2
  tag scope: id_FB=global, iq_FB=global
  wires:
  Gain_a/1 -> Mux_a/1
  in_1/1 -> Gain_a/1
  [cossin] -> Mux_a/2
  Mux_a/1 -> Fcn_a/1, Fcn_b/1
  Fcn_b/1 -> [iq_FB]
  Fcn_a/1 -> [id_FB]

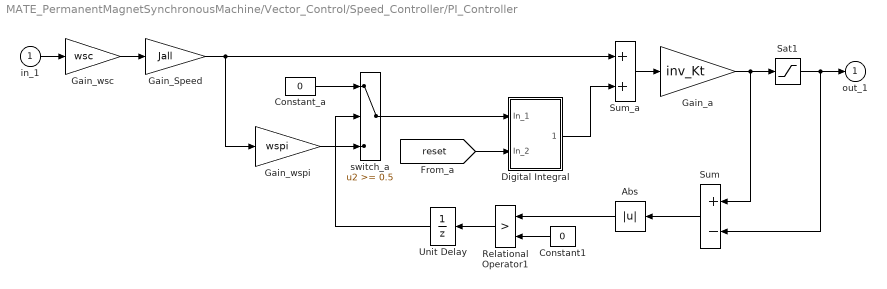
== system MATE_PermanentMagnetSynchronousMachine/Vector_Control/Speed_Controller/PI_Controller ==
  in_1 : Inport
  Abs : Abs  SaturateOnIntegerOverflow=off
  Constant1 : Constant  Value=0
  Constant_a : Constant  Value=0
  Digital Integral : Subsystem
      mask Display: disp(' 1 \n -- \n s ')
  Gain_Speed : Gain  Gain=Jall  SaturateOnIntegerOverflow=on  OutDataTypeStr=Inherit: Same as input  ParamDataTypeStr=Inherit: Same as input
  Gain_a : Gain  Gain=inv_Kt  SaturateOnIntegerOverflow=on  OutDataTypeStr=Inherit: Same as input  ParamDataTypeStr=Inherit: Same as input
  Gain_wsc : Gain  Gain=wsc  SaturateOnIntegerOverflow=on  OutDataTypeStr=Inherit: Same as input  ParamDataTypeStr=Inherit: Same as input
  Gain_wspi : Gain  Gain=wspi  SaturateOnIntegerOverflow=on  OutDataTypeStr=Inherit: Same as input  ParamDataTypeStr=Inherit: Same as input
  Relational Operator1 : RelationalOperator  Operator=>  InputSameDT=off
  Sat1 : Saturate  UpperLimit=iq_max  LowerLimit=-iq_max
  Sum : Sum  Inputs=+-  InputSameDT=on  SaturateOnIntegerOverflow=on  OutDataTypeStr=Inherit: Same as first input
  Sum_a : Sum  InputSameDT=on  SaturateOnIntegerOverflow=on  OutDataTypeStr=Inherit: Same as first input
  Unit Delay : UnitDelay  SampleTime=-1  HasFrameUpgradeWarning=on
  switch_a : Switch  Threshold=0.5
  out_1 : Outport
  wires:
  Gain_wspi/1 -> switch_a/3
  Gain_wsc/1 -> Gain_Speed/1
  in_1/1 -> Gain_wsc/1
  Constant_a/1 -> switch_a/1
  Gain_Speed/1 -> Gain_wspi/1, Sum_a/1
  switch_a/1 -> Digital Integral/1(In_1)
  [reset] -> Digital Integral/2(In_2)
  Digital Integral/1(Out_1) -> Sum_a/2
  Sum_a/1 -> Gain_a/1
  Gain_a/1 -> Sat1/1, Sum/1
  Constant1/1 -> Relational Operator1/2
  Sum/1 -> Abs/1
  Relational Operator1/1 -> Unit Delay/1
  Sat1/1 -> out_1/1, Sum/2
  Unit Delay/1 -> switch_a/2
  Abs/1 -> Relational Operator1/1

== system MATE_PermanentMagnetSynchronousMachine/Vector_Control/Speed_Controller/error ==
  in_1 : Inport
  in_2 : Inport  Port=2
  Mux_a : Mux  Inputs=2
  Sum_a : Sum  Inputs=+-  InputSameDT=on  SaturateOnIntegerOverflow=on  OutDataTypeStr=Inherit: Same as first input
  gain_a : Gain  Gain=rad_to_rpm  SaturateOnIntegerOverflow=on  OutDataTypeStr=Inherit: Same as input  ParamDataTypeStr=Inherit: Same as input
  out_1 : Outport
  tag scope: Mon_Wr=global
  wires:
  Sum_a/1 -> out_1/1
  in_2/1 -> Mux_a/2, Sum_a/2
  in_1/1 -> Sum_a/1, Mux_a/1
  Mux_a/1 -> gain_a/1
  gain_a/1 -> [Mon_Wr]

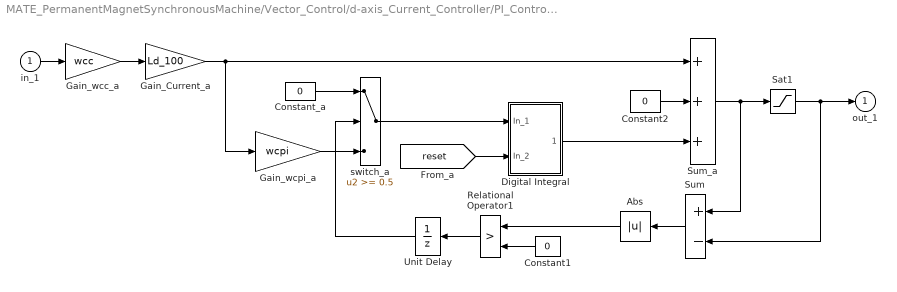
== system MATE_PermanentMagnetSynchronousMachine/Vector_Control/d-axis_Current_Controller/PI_Controller ==
  in_1 : Inport
  Abs : Abs  SaturateOnIntegerOverflow=off
  Constant1 : Constant  Value=0
  Constant2 : Constant  Value=0
  Constant_a : Constant  Value=0
  Digital Integral : Subsystem
      mask Display: disp(' 1 \n -- \n s ')
  Gain_Current_a : Gain  Gain=Ld_100  SaturateOnIntegerOverflow=on  OutDataTypeStr=Inherit: Same as input  ParamDataTypeStr=Inherit: Same as input
  Gain_wcc_a : Gain  Gain=wcc  SaturateOnIntegerOverflow=on  OutDataTypeStr=Inherit: Same as input  ParamDataTypeStr=Inherit: Same as input
  Gain_wcpi_a : Gain  Gain=wcpi  SaturateOnIntegerOverflow=on  OutDataTypeStr=Inherit: Same as input  ParamDataTypeStr=Inherit: Same as input
  Relational Operator1 : RelationalOperator  Operator=>  InputSameDT=off
  Sat1 : Saturate  UpperLimit=V_upper  LowerLimit=-V_upper
  Sum : Sum  Inputs=+-  InputSameDT=on  SaturateOnIntegerOverflow=on  OutDataTypeStr=Inherit: Same as first input
  Sum_a : Sum  Inputs=+++  InputSameDT=on  SaturateOnIntegerOverflow=on  OutDataTypeStr=Inherit: Same as first input
  Unit Delay : UnitDelay  SampleTime=-1  HasFrameUpgradeWarning=on
  switch_a : Switch  Threshold=0.5
  out_1 : Outport
  wires:
  [reset] -> Digital Integral/2(In_2)
  Gain_Current_a/1 -> Gain_wcpi_a/1, Sum_a/1
  Constant_a/1 -> switch_a/1
  Gain_wcc_a/1 -> Gain_Current_a/1
  in_1/1 -> Gain_wcc_a/1
  Digital Integral/1(Out_1) -> Sum_a/3
  Constant2/1 -> Sum_a/2
  Sum_a/1 -> Sat1/1, Sum/1
  switch_a/1 -> Digital Integral/1(In_1)
  Gain_wcpi_a/1 -> switch_a/3
  Constant1/1 -> Relational Operator1/2
  Sat1/1 -> out_1/1, Sum/2
  Sum/1 -> Abs/1
  Relational Operator1/1 -> Unit Delay/1
  Unit Delay/1 -> switch_a/2
  Abs/1 -> Relational Operator1/1

== system MATE_PermanentMagnetSynchronousMachine/Vector_Control/d-axis_Current_Controller/error ==
  in_1 : Inport
  in_2 : Inport  Port=2
  Mux_a : Mux  Inputs=2
  Sum_a : Sum  Inputs=+-  InputSameDT=on  SaturateOnIntegerOverflow=on  OutDataTypeStr=Inherit: Same as first input
  gain_a : Gain  Gain=inv_id_100*100  SaturateOnIntegerOverflow=on  OutDataTypeStr=Inherit: Same as input  ParamDataTypeStr=Inherit: Same as input
  out_1 : Outport
  tag scope: Mon_id=global
  wires:
  in_1/1 -> Sum_a/1, Mux_a/1
  in_2/1 -> Sum_a/2, Mux_a/2
  Sum_a/1 -> out_1/1
  Mux_a/1 -> gain_a/1
  gain_a/1 -> [Mon_id]

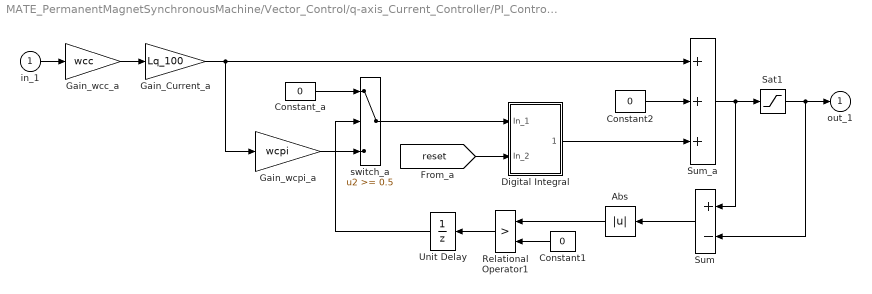
== system MATE_PermanentMagnetSynchronousMachine/Vector_Control/q-axis_Current_Controller/PI_Controller ==
  in_1 : Inport
  Abs : Abs  SaturateOnIntegerOverflow=off
  Constant1 : Constant  Value=0
  Constant2 : Constant  Value=0
  Constant_a : Constant  Value=0
  Digital Integral : Subsystem
      mask Display: disp(' 1 \n -- \n s ')
  Gain_Current_a : Gain  Gain=Lq_100  SaturateOnIntegerOverflow=on  OutDataTypeStr=Inherit: Same as input  ParamDataTypeStr=Inherit: Same as input
  Gain_wcc_a : Gain  Gain=wcc  SaturateOnIntegerOverflow=on  OutDataTypeStr=Inherit: Same as input  ParamDataTypeStr=Inherit: Same as input
  Gain_wcpi_a : Gain  Gain=wcpi  SaturateOnIntegerOverflow=on  OutDataTypeStr=Inherit: Same as input  ParamDataTypeStr=Inherit: Same as input
  Relational Operator1 : RelationalOperator  Operator=>  InputSameDT=off
  Sat1 : Saturate  UpperLimit=V_upper  LowerLimit=-V_upper
  Sum : Sum  Inputs=+-  InputSameDT=on  SaturateOnIntegerOverflow=on  OutDataTypeStr=Inherit: Same as first input
  Sum_a : Sum  Inputs=+++  InputSameDT=on  SaturateOnIntegerOverflow=on  OutDataTypeStr=Inherit: Same as first input
  Unit Delay : UnitDelay  SampleTime=-1  HasFrameUpgradeWarning=on
  switch_a : Switch  Threshold=0.5
  out_1 : Outport
  wires:
  Constant2/1 -> Sum_a/2
  Digital Integral/1(Out_1) -> Sum_a/3
  in_1/1 -> Gain_wcc_a/1
  Gain_wcc_a/1 -> Gain_Current_a/1
  Constant_a/1 -> switch_a/1
  Gain_Current_a/1 -> Gain_wcpi_a/1, Sum_a/1
  [reset] -> Digital Integral/2(In_2)
  Sum_a/1 -> Sat1/1, Sum/1
  switch_a/1 -> Digital Integral/1(In_1)
  Gain_wcpi_a/1 -> switch_a/3
  Constant1/1 -> Relational Operator1/2
  Sum/1 -> Abs/1
  Relational Operator1/1 -> Unit Delay/1
  Sat1/1 -> out_1/1, Sum/2
  Unit Delay/1 -> switch_a/2
  Abs/1 -> Relational Operator1/1

== system MATE_PermanentMagnetSynchronousMachine/Vector_Control/q-axis_Current_Controller/error ==
  in_1 : Inport
  in_2 : Inport  Port=2
  Mux_a : Mux  Inputs=2
  Sum_a : Sum  Inputs=+-  InputSameDT=on  SaturateOnIntegerOverflow=on  OutDataTypeStr=Inherit: Same as first input
  gain_a : Gain  Gain=inv_iq_100*100  SaturateOnIntegerOverflow=on  OutDataTypeStr=Inherit: Same as input  ParamDataTypeStr=Inherit: Same as input
  out_1 : Outport
  tag scope: Mon_iq=global
  wires:
  gain_a/1 -> [Mon_iq]
  Mux_a/1 -> gain_a/1
  Sum_a/1 -> out_1/1
  in_2/1 -> Mux_a/2, Sum_a/2
  in_1/1 -> Sum_a/1, Mux_a/1

== system MATE_PermanentMagnetSynchronousMachine/Vector_Control/Speed_Controller/PI_Controller/Digital Integral ==
  In_1 : Inport
  In_2 : Inport  Port=2
  Constant : Constant  Value=0
  Gain_a : Gain  Gain=Tsc  SaturateOnIntegerOverflow=on  OutDataTypeStr=Inherit: Same as input  ParamDataTypeStr=Inherit: Same as input
  Sum_a : Sum  InputSameDT=on  SaturateOnIntegerOverflow=on  OutDataTypeStr=Inherit: Same as first input
  Switch_a : Switch  Threshold=0.5
  Unit Delay_a : UnitDelay  SampleTime=-1  HasFrameUpgradeWarning=on
  Out_1 : Outport
  wires:
  Unit Delay_a/1 -> Sum_a/2
  Constant/1 -> Switch_a/3
  In_1/1 -> Gain_a/1
  Gain_a/1 -> Sum_a/1
  Sum_a/1 -> Switch_a/1
  Switch_a/1 -> Unit Delay_a/1, Out_1/1
  In_2/1 -> Switch_a/2

== system MATE_PermanentMagnetSynchronousMachine/Vector_Control/d-axis_Current_Controller/PI_Controller/Digital Integral ==
  In_1 : Inport
  In_2 : Inport  Port=2
  Constant : Constant  Value=0
  Gain_a : Gain  Gain=Tsc  SaturateOnIntegerOverflow=on  OutDataTypeStr=Inherit: Same as input  ParamDataTypeStr=Inherit: Same as input
  Sum_a : Sum  InputSameDT=on  SaturateOnIntegerOverflow=on  OutDataTypeStr=Inherit: Same as first input
  Switch_a : Switch  Threshold=0.5
  Unit Delay_a : UnitDelay  SampleTime=-1  HasFrameUpgradeWarning=on
  Out_1 : Outport
  wires:
  Unit Delay_a/1 -> Sum_a/2
  Constant/1 -> Switch_a/3
  In_1/1 -> Gain_a/1
  Gain_a/1 -> Sum_a/1
  Sum_a/1 -> Switch_a/1
  Switch_a/1 -> Unit Delay_a/1, Out_1/1
  In_2/1 -> Switch_a/2

== system MATE_PermanentMagnetSynchronousMachine/Vector_Control/q-axis_Current_Controller/PI_Controller/Digital Integral ==
  In_1 : Inport
  In_2 : Inport  Port=2
  Constant : Constant  Value=0
  Gain_a : Gain  Gain=Tsc  SaturateOnIntegerOverflow=on  OutDataTypeStr=Inherit: Same as input  ParamDataTypeStr=Inherit: Same as input
  Sum_a : Sum  InputSameDT=on  SaturateOnIntegerOverflow=on  OutDataTypeStr=Inherit: Same as first input
  Switch_a : Switch  Threshold=0.5
  Unit Delay_a : UnitDelay  SampleTime=-1  HasFrameUpgradeWarning=on
  Out_1 : Outport
  wires:
  Unit Delay_a/1 -> Sum_a/2
  Constant/1 -> Switch_a/3
  In_1/1 -> Gain_a/1
  Gain_a/1 -> Sum_a/1
  Sum_a/1 -> Switch_a/1
  Switch_a/1 -> Unit Delay_a/1, Out_1/1
  In_2/1 -> Switch_a/2
